simulink model "PN_generator_RxV2"  (R2020a)
settings: Solver=VariableStepAuto  StartTime=0.0  StopTime=inf  RelTol=1e-3
undefined symbols (not defined in the file): Fs, ip, usb
libraries: commfilt2 x2, plutoradiolib x1, commdigbbndpm3 x1
settings Model: Creator=juanj  LastModifiedBy=juanj

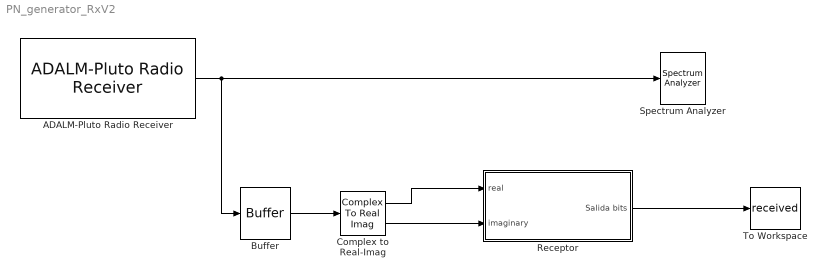
== system PN_generator_RxV2 ==
  ADALM-Pluto Radio Receiver : plutoradiolib/ADALM-Pluto Radio Receiver  RadioID=usb:1  uri=ip:10.0.0.200  CenterFrequencySource=Dialog  CenterFrequency=900e6  GainSource=AGC Slow Attack  GainSourceBlock=AGC Slow Attack  Gain=10  ChannelMapping=1  BasebandSampleRate=500e3  OutputDataType=single  SamplesPerFrame=2128  OverflowOutputPort=off  EnableBurstMode=off  NumFramesInBurst=1  ShowAdvancedProperties=off  UseCustomFilter=off  filtPathRates=[737280000 11520000 3840000 1920000 960000 240000]  filtCoefficients=[-192 82 85 -215 228 -102 -110 290 -318 145 160 -426 471 -215 -238 633 -697 318 349 -923 1009 -457 -498 1309 -1423 640 693 -1812 1959 -876 -945 2458 -2647 1180 1268 -3290 3534 -1572 -1688 4375 -4698 2091 2247 -5836 6284 -2807 -3031 7918 -8588 3870 4225 -11182 12324 -5662 -6330 17255 -19735 9507 11312 -33568 43355 -25227 -42139 305542 305542 -42139 -25227 43355 -33568 11312 9507 -19735 17255 -6330 -5662 12324 -11182 4225 3870 -8588 7918 -3031 -2807 6284 -5836 2247 2091 -4698 4375 -1688 -1572 3534 -3290 1268 1180 -2647 2458 -945 -876 1959 -1812 693 640 -1423 1309 -498 -457 1009 -923 349 318 -697 633 -238 -215 471 -426 160 145 -318 290 -110 -102 228 -215 85 82 -192]  filtCoefficientSize=128  filtDecimInterpFactor=4  filtGain=-12  filtRFBandwidth=18000000  filterConfigStruct=struct()  EnableQuadratureCorrection=on  EnableRFDCCorrection=on  EnableBasebandDCCorrection=on  FrequencyCorrection=0  OverrideSampleTime=off  SampleTime=0.02  DataTimeout=Inf  ENSMPinControlMode=None  BISTLoopbackMode=Disabled  BISTToneInject=Disabled  BISTSignalGen=PRBS  BISTToneFreq=Fs/32  BISTToneLevel=0
      settings: SourceProductBaseCode=PLUTO
  Buffer : Buffer  N=1  OutputFrames=off
  Complex to Real-Imag : ComplexToRealImag
  Receptor : Subsystem
  Spectrum Analyzer : SpectrumAnalyzer
  To Workspace : ToWorkspace  VariableName=received  SampleTime=1/10000
      settings: Save2DSignal=2-D array (concatenate along first dimension)
  wires:
  ADALM-Pluto Radio Receiver/1 -> Buffer/1, Spectrum Analyzer/1
  Complex to Real-Imag/2 -> Receptor/2(imaginary)
  Complex to Real-Imag/1 -> Receptor/1(real)
  Receptor/1(Salida bits) -> To Workspace/1
  Buffer/1 -> Complex to Real-Imag/1

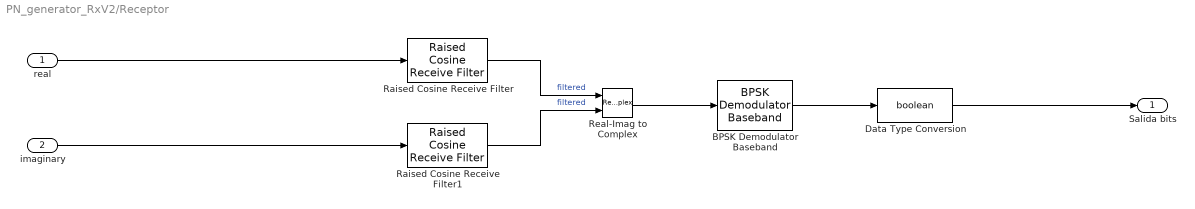
== system PN_generator_RxV2/Receptor ==
  real : Inport
  imaginary : Inport  Port=2
  BPSK Demodulator Baseband : commdigbbndpm3/BPSK Demodulator Baseband  DecType=Hard decision  VarSource=Dialog  Variance=1  Ph=0  outDtype=Inherit via internal rule  derotateFactorWordLen=16  derotateFactorDataTypeStr=Inherit: Same word length as input  derotateFactorLastDataTypeStr=Inherit: Same word length as input
  Data Type Conversion : DataTypeConversion  OutDataTypeStr=boolean
  Raised Cosine Receive Filter : commfilt2/Raised Cosine Receive Filter  filtType=Square root  R=0.5  filtSpan=16  N=16  downFactor=16  downOffset=0  filterGain=2  RateOptions=Allow multirate processing  framing=Mute  checkCoeff=off  variableName=rcRxFilt  currentFiltSpan=16  D=(16)/2  inputOffset=0  sampMode=Mute  saveAsFlag=0  rateMode=Downsampling  checkGain=Normalized  launchFVT=on  roundingMode=Floor  overflowMode=off  coeffDataTypeStr=Inherit: Same word length as input  coeffMin=[]  coeffMax=[]  coeffLastDataTypeStr=Inherit: Same word length as input  accumDataTypeStr=Inherit: Same as product output  accumLastDataTypeStr=Inherit: Same as product output  outputDataTypeStr=Inherit: Same as accumulator  outputMin=[]  outputMax=[]  outputLastDataTypeStr=Inherit: Same as accumulator
  Raised Cosine Receive Filter1 : commfilt2/Raised Cosine Receive Filter  filtType=Square root  R=0.5  filtSpan=16  N=16  downFactor=16  downOffset=0  filterGain=2  RateOptions=Allow multirate processing  framing=Mute  checkCoeff=off  variableName=rcRxFilt1  currentFiltSpan=16  D=(16)/2  inputOffset=0  sampMode=Mute  saveAsFlag=0  rateMode=Downsampling  checkGain=Normalized  launchFVT=on  roundingMode=Floor  overflowMode=off  coeffDataTypeStr=Inherit: Same word length as input  coeffMin=[]  coeffMax=[]  coeffLastDataTypeStr=Inherit: Same word length as input  accumDataTypeStr=Inherit: Same as product output  accumLastDataTypeStr=Inherit: Same as product output  outputDataTypeStr=Inherit: Same as accumulator  outputMin=[]  outputMax=[]  outputLastDataTypeStr=Inherit: Same as accumulator
  Real-Imag to Complex : RealImagToComplex
  Salida bits : Outport
  wires:
  Raised Cosine Receive Filter/1 -> Real-Imag to Complex/1  "filtered"
  BPSK Demodulator Baseband/1 -> Data Type Conversion/1
  imaginary/1 -> Raised Cosine Receive Filter1/1
  Raised Cosine Receive Filter1/1 -> Real-Imag to Complex/2  "filtered"
  Real-Imag to Complex/1 -> BPSK Demodulator Baseband/1
  real/1 -> Raised Cosine Receive Filter/1
  Data Type Conversion/1 -> Salida bits/1
